simulink model "bruit_TD2"  (R2024a)
settings: Solver=ode45  StartTime=0.0  StopTime=t_sim  RelTol=1e-3  EnableMultiTasking=on
values from neighbouring files (symbols this model uses):
  ts = 0.000001    (= 1e-06)    [main.m]
libraries: simulink x1
settings Model: Creator=mailly  LastModifiedBy=diogo.klafke-ogochi
settings SolverCC: AlgebraicLoopSolver=TrustRegion
settings DataIOCC: LimitDataPoints=on  SaveFormat=Array  SignalLoggingSaveFormat=ModelDataLogs  ReturnWorkspaceOutputs=off
settings OptimizationCC: InitFltsAndDblsToZero=on  LifeSpan=inf
settings DebuggingCC: SaveWithParameterizedLinksMsg=none  UnderspecifiedInitializationDetection=Classic  MergeDetectMultiDrivingBlocksExec=none  SignalResolutionControl=TryResolveAllWithWarning  SolverPrmCheckMsg=warning  MultiTaskDSMMsg=warning  MultiTaskCondExecSysMsg=none  FcnCallInpInsideContextMsg=warning  UnconnectedInputMsg=warning  UnconnectedOutputMsg=warning  UnconnectedLineMsg=warning  AllowSymbolicDim=off  SFUnexpectedBacktrackingDiag=warning  SFNoUnconditionalDefaultTransitionDiag=warning  SFExecutionAtInitializationDiag=none  ArithmeticOperatorsInVariantConditions=warning
settings HardwareCC: ProdBitPerPointer=32  ProdBitPerSizeT=32  ProdBitPerPtrDiffT=32  ProdLargestAtomicFloat=None  ProdIntDivRoundTo=Undefined  ProdEndianess=Unspecified  ProdWordSize=32  ProdHWDeviceType=32-bit Generic
settings ModelReferenceCC: EnableRefExpFcnMdlSchedulingChecks=on  PropagateSignalLabelsOutOfModel=off
settings SFSimCC: SimUseLocalCustomCode=off  CustomCodeUndefinedFunction=UseInterfaceOnly
settings RTWCC: RTWUseLocalCustomCode=off  GPUComputeCapability=3.5
settings CodeAppCC: StateflowObjectComments=on
settings GRTTargetCC: TargetFcnLib=ansi_tfl_tmw.mat  TargetLangStandard=C89/C90 (ANSI)  CombineOutputUpdateFcns=off  GRTInterface=on
settings ConfigComp: CovMetricSettings=dw  CovSaveCumulativeToWorkspaceVar=on  CovSaveSingleToWorkspaceVar=on  CovExternalEMLEnable=off

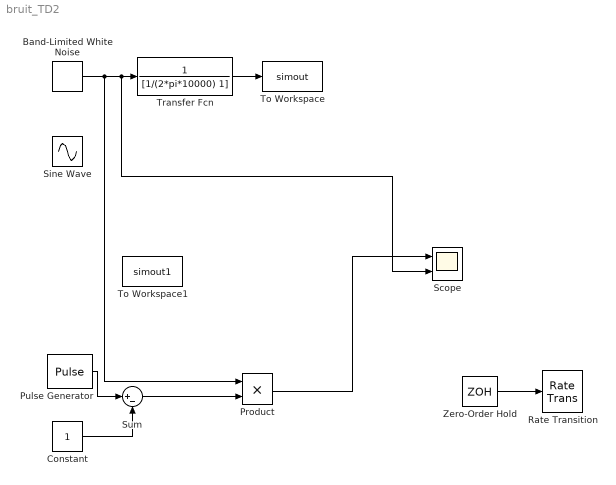
== system bruit_TD2 ==
  Band-Limited White Noise : simulink/Sources/Band-Limited White Noise  Cov=[0.5*10^-16]  Ts=ts  seed=[23341]
  Constant : Constant
  Product : Product  RndMeth=Zero  SampleTime=0
  Pulse Generator : DiscretePulseGenerator  PulseType=Time based  Amplitude=2  Period=1/20  PulseWidth=50
  Rate Transition : RateTransition
  Scope : Scope  NumInputPorts=2
  Sine Wave : Sin  Amplitude=1e-6  Frequency=2*pi*10  SampleTime=0
  Sum : Sum  Inputs=|+-
  To Workspace : ToWorkspace  VariableName=simout  SampleTime=ts
  To Workspace1 : ToWorkspace  VariableName=simout1  SampleTime=ts
  Transfer Fcn : TransferFcn  Denominator=[1/(2*pi*10000) 1]
  Zero-Order Hold : ZeroOrderHold  SampleTime=1/200
  wires:
  Constant/1 -> Sum/2
  Pulse Generator/1 -> Sum/1
  Sum/1 -> Product/2
  Zero-Order Hold/1 -> Rate Transition/1
  Band-Limited White Noise/1 -> Product/1, Scope/2, Transfer Fcn/1
  Transfer Fcn/1 -> To Workspace/1
  Product/1 -> Scope/1
